simulink model "GcFilterTest"  (R2024a)
settings: Solver=VariableStepAuto  StartTime=0.0  StopTime=0.3  RelTol=1e-3
undefined symbols (not defined in the file or in its folder): vr, wg
libraries: cstblocks x4
settings Model: Creator=FactCore  LastModifiedBy=FactCore

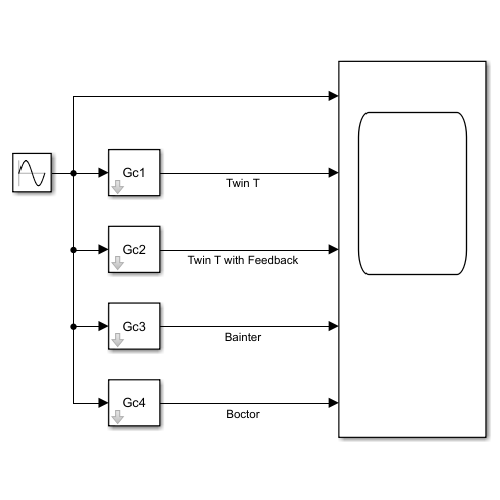
[thumbnail: Simulink's stored preview of the top-level diagram]
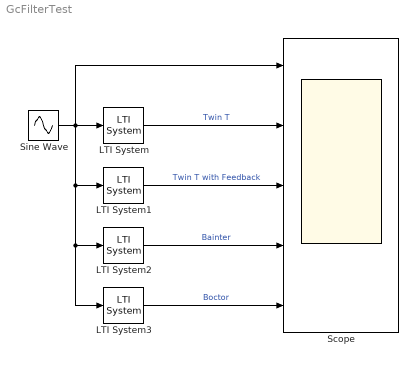
== system GcFilterTest ==
  LTI System : cstblocks/LTI System  sys=Gc1  IC=[]  PadeOrder=0
  LTI System1 : cstblocks/LTI System  sys=Gc2  IC=[]  PadeOrder=0
  LTI System2 : cstblocks/LTI System  sys=Gc3  IC=[]  PadeOrder=0
  LTI System3 : cstblocks/LTI System  sys=Gc4  IC=[]  PadeOrder=0
  Scope : Scope  NumInputPorts=5
  Sine Wave : Sin  Amplitude=vr*sqrt(2)  Frequency=wg  SampleTime=0
  wires:
  Sine Wave/1 -> LTI System3/1, LTI System2/1, LTI System1/1, Scope/1, LTI System/1
  LTI System/1 -> Scope/2  "Twin T"
  LTI System1/1 -> Scope/3  "Twin T with Feedback"
  LTI System2/1 -> Scope/4  "Bainter"
  LTI System3/1 -> Scope/5  "Boctor"
